simulink model "FLV_simulink_3_21"  (R2021b)
settings: Solver=FixedStepAuto  StartTime=0.0  StopTime=10.0  FixedStep=0.01  RelTol=1e-3
values from neighbouring files (symbols this model uses):
  flaCurve = [-15 -5 0 0.401 0.402 0.4035 0.52725 0.62875 0.71875 0.86125 1.045 1.2175 ... (38 elements, 19x2)]    [force_curves.mat]
  fLenCurve = [ls2, fl_int(:,1)]    [load_data.m]
  flpCurve = [-15 -5 0.998 0.999 1 1.1 1.2 1.3 1.4 1.5 1.6 1.601 ... (30 elements, 15x2)]    [force_curves.mat]
  fvCurve = [-1 -0.95 -0.9 -0.85 -0.8 -0.75 -0.7 -0.65 -0.6 -0.55 -0.5 -0.45 ... (82 elements, 41x2)]    [force_curves.mat]    (also in load_data.m = [-ls, fv_int])
undefined symbols (not defined in the file or in its folder): fvCurve2
libraries: simulink x1
settings Model: Creator=rauf  LastModifiedBy=rauf
settings SolverCC: AlgebraicLoopSolver=TrustRegion
settings DebuggingCC: SFMachineParentedDataDiag=warning

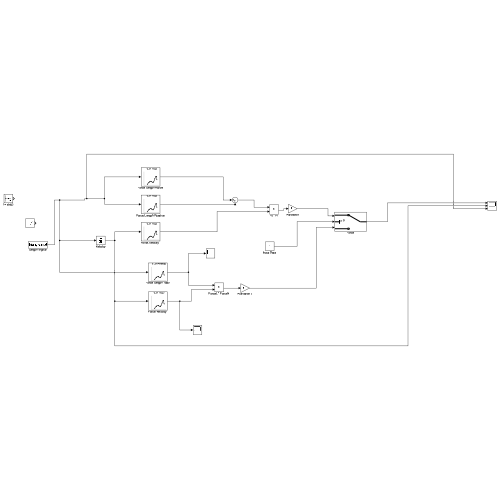
[thumbnail: Simulink's stored preview of the top-level diagram]
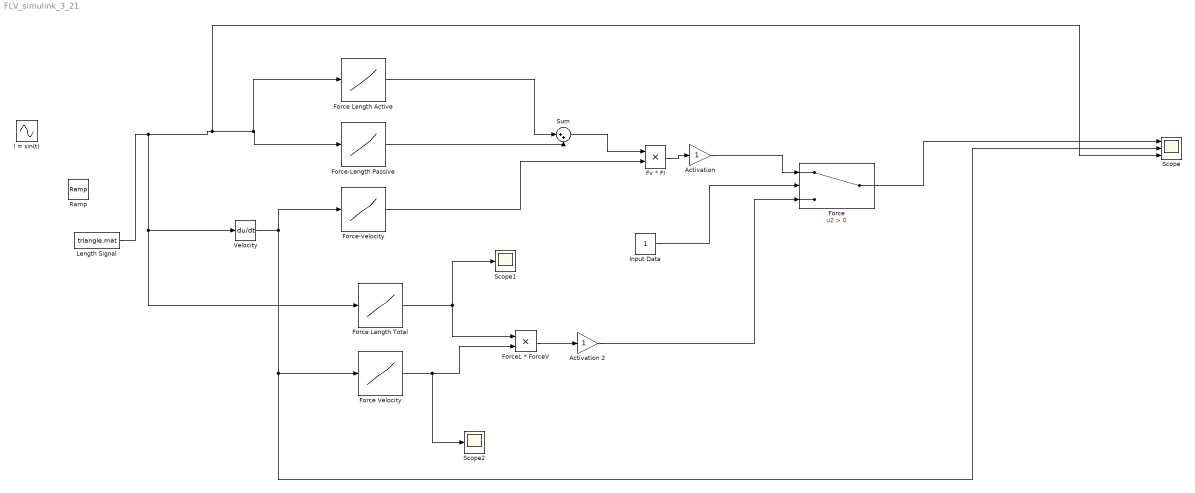
== system FLV_simulink_3_21 ==
  Activation : Gain
  Activation 2 : Gain
  Force : Switch  Criteria=u2 > Threshold
  Force Length Active : Lookup_n-D  NumberOfTableDimensions=1  BreakpointsForDimension1=flaCurve(:,1)  Table=flaCurve(:,2)  InterpMethod=Cubic spline  InternalRulePriority=Speed  RndMeth=Simplest  InputSameDT=on
  Force Length Total : Lookup_n-D  NumberOfTableDimensions=1  BreakpointsForDimension1=fLenCurve(:,1)  Table=fLenCurve(:,2)  InterpMethod=Akima spline  InternalRulePriority=Speed  RndMeth=Simplest  InputSameDT=on
  "Force Velocity " : Lookup_n-D  NumberOfTableDimensions=1  BreakpointsForDimension1=fvCurve2(:,1)  Table=fvCurve2(:,2)  InterpMethod=Cubic spline  InternalRulePriority=Speed  RndMeth=Simplest  InputSameDT=on
  Force-Length Passive : Lookup_n-D  NumberOfTableDimensions=1  BreakpointsForDimension1=flpCurve(:,1)  Table=flpCurve(:,2)  InterpMethod=Cubic spline  InternalRulePriority=Speed  RndMeth=Simplest  InputSameDT=on
  "Force-velocity " : Lookup_n-D  NumberOfTableDimensions=1  BreakpointsForDimension1=fvCurve(:,1)  Table=fvCurve(:,2)  InterpMethod=Cubic spline  InternalRulePriority=Speed  RndMeth=Simplest  InputSameDT=on
  ForceL * ForceV : Product
  Fv * Fl : Product
  Input Data : Constant
  Length Signal : FromFile  FileName=triangle.mat  SampleTime=0
  Ramp : simulink/Sources/Ramp  slope=1  start=0  InitialOutput=0
  Scope : Scope  NumInputPorts=3
  Scope1 : Scope
  Scope2 : Scope
  Sum : Sum  Inputs=|++
  Velocity : Derivative
  l = sin(t) : Sin  SampleTime=0
  wires:
  Length Signal/1 -> Velocity/1, Force Length Total/1, Scope/3, Force-Length Passive/1, Force Length Active/1
  Force-Length Passive/1 -> Sum/2
  Velocity/1 -> Scope/2, "Force Velocity "/1, "Force-velocity "/1
  "Force-velocity "/1 -> Fv * Fl/2
  Sum/1 -> Fv * Fl/1
  Force Length Active/1 -> Sum/1
  Fv * Fl/1 -> Activation/1
  Activation/1 -> Force/1
  Input Data/1 -> Force/2
  Force/1 -> Scope/1
  Force Length Total/1 -> Scope1/1, ForceL * ForceV/1
  "Force Velocity "/1 -> Scope2/1, ForceL * ForceV/2
  ForceL * ForceV/1 -> Activation 2/1
  Activation 2/1 -> Force/3
